simulink model "hierarchical_controller"  (R2025b)
settings: Solver=VariableStepAuto  StartTime=0.0  StopTime=30.0  RelTol=1e-3
InitFcn:
  | %% INITIALIZATION
  | 
  | clearvars -except out
  | clc
  | 
  | %% UAV PARAMETERS
  | 
  | mass = 1.2;        % [kg] mass used by controllers
  | mass_real = 1.2;  % [kg] mass used by dynamics
  | 
  | Ib = diag([1.2416 1.2416 2*1.2416]);
  | Ib_ctrl = diag([1.0 0.85 1.80]);
  | %Ib_ctrl = diag([1.2416 1.2416 2*1.2416]);
  | %% SAMPLING TIME
  | 
  | Ts = 0.001;
  | 
  | %% PLANNER
  | 
  | t_iniz = 0;
  | ttot = 22;       % trajectory duration [s]
  | tdead = 8;       % final steady-state time [s]
  | tot_time = ttot + tdead;
  | 
  | % Include exactly t = ttot
  | t1 = 0:Ts:ttot;
  | t_dead = (ttot+Ts):Ts:tot_time;
  | t = [t1, t_dead];
  | 
  | N1 = length(t1);
  | Ndead = length(t_dead);
  | 
  | %% INITIAL CONDITIONS
  | 
  | x0 = 0;
  | y0 = 0;
  | z0 = -1;
  | psi0 = 0;
  | 
  | x0_real = x0;
  | y0_real = y0;
  | z0_real = z0;
  | 
  | pos_0 = [x0_real y0_real z0_real];
  | lin_vel_0 = [0 0 0];
  | w_bb_0 = [0 0 0];
  | 
  | %% SMOOTH NORMALIZED TIME
  | 
  | sigma = t1 / ttot;
  | 
  | % 7th-order smooth step:
  | % s(0)=0, s(1)=1
  | % sdot(0)=sdot(1)=0
  | % sddot(0)=sddot(1)=0
  | % sdddot(0)=sdddot(1)=0
  | 
  | s = 35*sigma.^4 - 84*sigma.^5 + 70*sigma.^6 - 20*sigma.^7;
  | 
  | sdot = (140*sigma.^3 ...
  |       - 420*sigma.^4 ...
  |       + 420*sigma.^5 ...
  |       - 140*sigma.^6) / ttot;
  | 
  | sddot = (420*sigma.^2 ...
  |        - 1680*sigma.^3 ...
  |        + 2100*sigma.^4 ...
  |        - 840*sigma.^5) / ttot^2;
  | 
  | %% DESIRED TRAJECTORY PARAMETERS
  | 
  | Dx = 1.20;
  | Dy = 0.70;
  | Dz = -1.70;
  | 
  | Ay_bump = 0.35;
  | Az_bump = 0.18;
  | 
  | psi_final = deg2rad(25);
  | psi_bump  = deg2rad(6);
  | 
  | %% DESIRED POSITION
  | 
  | x_d = x0 + Dx*s;
  | 
  | y_d = y0 + Dy*s + Ay_bump*sin(2*pi*s);
  | 
  | z_d = z0 + Dz*s + Az_bump*sin(pi*s);
  | 
  | psi_d_traj = psi0 + psi_final*s + psi_bump*sin(pi*s);
  | 
  | %% DERIVATIVES WITH RESPECT TO s
  | 
  | x_s = Dx;
  | x_ss = 0;
  | 
  | y_s = Dy + Ay_bump*2*pi*cos(2*pi*s);
  | y_ss = -Ay_bump*(2*pi)^2*sin(2*pi*s);
  | 
  | z_s = Dz + Az_bump*pi*cos(pi*s);
  | z_ss = -Az_bump*pi^2*sin(pi*s);
  | 
  | psi_s = psi_final + psi_bump*pi*cos(pi*s);
  | psi_ss = -psi_bump*pi^2*sin(pi*s);
  | 
  | %% DESIRED VELOCITY
  | 
  | dot_x_d = x_s .* sdot;
  | dot_y_d = y_s .* sdot;
  | dot_z_d = z_s .* sdot;
  | 
  | dot_psi_d_traj = psi_s .* sdot;
  | 
  | %% DESIRED ACCELERATION
  | 
  | ddot_x_d = x_ss .* sdot.^2 + x_s .* sddot;
  | ddot_y_d = y_ss .* sdot.^2 + y_s .* sddot;
  | ddot_z_d = z_ss .* sdot.^2 + z_s .* sddot;
  | 
  | ddot_psi_d_traj = psi_ss .* sdot.^2 + psi_s .* sddot;
  | 
  | %% ADD FINAL STEADY-STATE PART
  | 
  | x_final = x_d(end);
  | y_final = y_d(end);
  | z_final = z_d(end);
  | psi_final_value = psi_d_traj(end);
  | 
  | p_d = zeros(4, length(t));
  | dot_p_d = zeros(4, length(t));
  | ddot_p_d = zeros(4, length(t));
  | 
  | p_d(1,:) = [x_d, x_final*ones(1, Ndead)];
  | p_d(2,:) = [y_d, y_final*ones(1, Ndead)];
  | p_d(3,:) = [z_d, z_final*ones(1, Ndead)];
  | p_d(4,:) = [psi_d_traj, psi_final_value*ones(1, Ndead)];
  | 
  | dot_p_d(1,:) = [dot_x_d, zeros(1, Ndead)];
  | dot_p_d(2,:) = [dot_y_d, zeros(1, Ndead)];
  | dot_p_d(3,:) = [dot_z_d, zeros(1, Ndead)];
  | dot_p_d(4,:) = [dot_psi_d_traj, zeros(1, Ndead)];
  | 
  | ddot_p_d(1,:) = [ddot_x_d, zeros(1, Ndead)];
  | ddot_p_d(2,:) = [ddot_y_d, zeros(1, Ndead)];
  | ddot_p_d(3,:) = [ddot_z_d, zeros(1, Ndead)];
  | ddot_p_d(4,:) = [ddot_psi_d_traj, zeros(1, Ndead)];
  | 
  | %% DATA FOR SIMULINK
  | 
  | csi_d = p_d(1:3,:);
  | dot_csi_d = dot_p_d(1:3,:);
  | ddot_csi_d = ddot_p_d(1:3,:);
  | 
  | psi_d = p_d(4,:);
  | dot_psi_d = dot_p_d(4,:);
  | ddot_psi_d = ddot_p_d(4,:);
  | 
  | %% DESIRED BODY X-AXIS FROM YAW
  | 
  | xb_des = zeros(3, length(t));
  | 
  | xb_des(1,:) = cos(psi_d);
  | xb_des(2,:) = sin(psi_d);
  | xb_des(3,:) = zeros(1, length(t));
  | 
  | %% EXTERNAL FORCE DISTURBANCE
  | 
  | f_ext = zeros(length(t), 3);
  | 
  | t_f_on = 8;
  | t_f_off = 14;
  | 
  | f_ex_amp = 1.0;    % [N]
  | f_ey_amp = 1.0;    % [N]
  | f_ez_amp = 0.0;    % [N]
  | 
  | t_smooth_f = 0.3;  % [s] smoothing time
  | 
  | w_on_f  = 0.5 * (1 + tanh((t - t_f_on)/t_smooth_f));
  | w_off_f = 0.5 * (1 - tanh((t - t_f_off)/t_smooth_f));
  | 
  | dist_window_f = w_on_f .* w_off_f;
  | 
  | f_ext(:,1) = f_ex_amp * dist_window_f(:);
  | f_ext(:,2) = f_ey_amp * dist_window_f(:);
  | f_ext(:,3) = f_ez_amp * dist_window_f(:);
  | 
  | f_ext_ts = timeseries(f_ext, t(:));
  | 
  | %% EXTERNAL TORQUE DISTURBANCE
  | 
  | tau_ext = zeros(length(t), 3);
  | 
  | t_tau_on = 8;
  | t_tau_off = 14;
  | 
  | tau_ex_amp = 0.0;    % [Nm]
  | tau_ey_amp = 0.5;    % [Nm]
  | tau_ez_amp = 0.0;    % [Nm]
  | 
  | t_smooth_tau = 0.3;  % [s] smoothing time
  | 
  | w_on_tau  = 0.5 * (1 + tanh((t - t_tau_on)/t_smooth_tau));
  | w_off_tau = 0.5 * (1 - tanh((t - t_tau_off)/t_smooth_tau));
  | 
  | dist_window_tau = w_on_tau .* w_off_tau;
  | 
  | tau_ext(:,1) = tau_ex_amp * dist_window_tau(:);
  | tau_ext(:,2) = tau_ey_amp * dist_window_tau(:);
  | tau_ext(:,3) = tau_ez_amp * dist_window_tau(:);
  | 
  | tau_ext_ts = timeseries(tau_ext, t(:));
  | 
  | 
  | %% CHECK
  | 
  | disp("InitFcn completed.")
  | disp("mass = " + string(mass) + " kg")
  | disp("mass_real = " + string(mass_real) + " kg")
  | disp("Simulation time = " + string(tot_time) + " s")
  | disp("Force disturbance: [" + string(f_ex_amp) + ", " + string(f_ey_amp) + ", " + string(f_ez_amp) + "] N")
  | disp("Torque disturbance: [" + string(tau_ex_amp) + ", " + string(tau_ey_amp) + ", " + string(tau_ez_amp) + "] Nm")
libraries: robotcorelib x1
settings Model: Creator=fabioruggiero  LastModifiedBy=miche
settings ModelReferenceCC: EnableRefExpFcnMdlSchedulingChecks=on
settings RTWCC: GPUComputeCapability=3.5

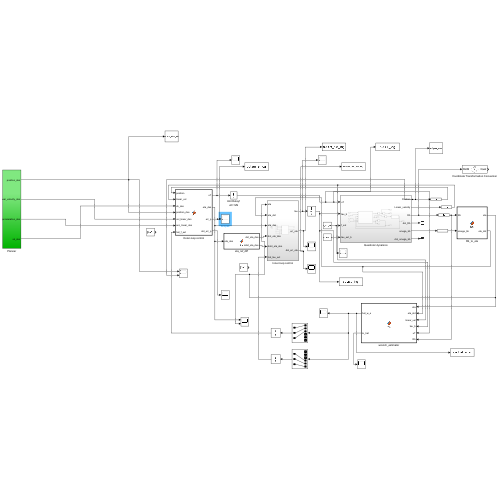
[thumbnail: Simulink's stored preview of the top-level diagram]
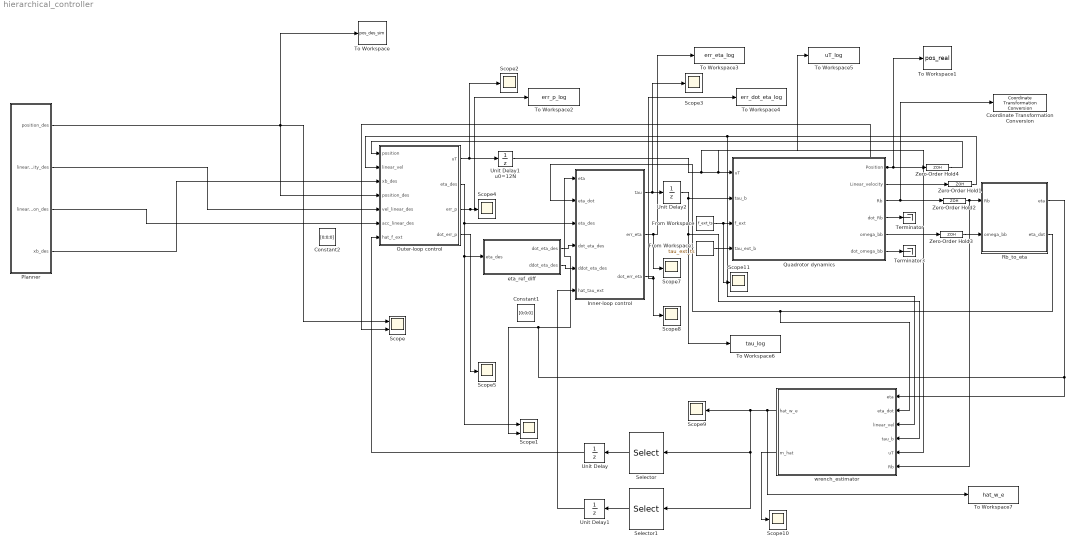
== system hierarchical_controller ==
  Constant1 : Constant  Value=[0;0;0]
  Constant2 : Constant  Value=[0;0;0]
  Coordinate Transformation Conversion : robotcorelib/Coordinate Transformation Conversion  InputRepresentation=Rotation Matrix  InputEulerSequence=ZYX  ShowTrVecInputPort=on  OutputRepresentation=Quaternion  OutputEulerSequence=ZYX  ShowTrVecOutputPort=on  SimulateUsing=Interpreted execution
  From Workspace : FromWorkspace  VariableName=f_ext_ts
  From Workspace1 : FromWorkspace  VariableName=tau_ext_ts
  Inner-loop control : Subsystem
  Outer-loop control : MATLAB Function  TreatAsAtomicUnit=on
  Planner : Subsystem
  Quadrotor dynamics : Subsystem
  Rb_to_eta : MATLAB Function  TreatAsAtomicUnit=on
  Scope : Scope  NumInputPorts=2
      settings: ActiveDisplayYMinimum=-4.8250002447828013  ActiveDisplayYMaximum=3.4250000522047972
  Scope1 : Scope  NumInputPorts=2
      settings: ActiveDisplayYMinimum=-1  ActiveDisplayYMaximum=1
  Scope{2..5,7..11} (9 alike) : Scope
      Scope10 settings: ActiveDisplayYMinimum=1.0530751929618971  ActiveDisplayYMaximum=1.5207401244876457  DataLoggingVariableName=ScopeData11
      Scope11 settings: ActiveDisplayYMinimum=-1  ActiveDisplayYMaximum=1  DataLoggingVariableName=ScopeData12
      Scope2 settings: ActiveDisplayYMinimum=-1  ActiveDisplayYMaximum=1  DataLoggingVariableName=ScopeData2
      Scope3 settings: ActiveDisplayYMinimum=-835.01616147047889  ActiveDisplayYMaximum=458.79322442296439  DataLoggingVariableName=ScopeData3
      Scope4 settings: ActiveDisplayYMinimum=-0.020825285520524945  ActiveDisplayYMaximum=0.020902843774846348  DataLoggingVariableName=ScopeData5
      Scope5 settings: ActiveDisplayYMinimum=-0.31823529054964583  ActiveDisplayYMaximum=0.47295316972389595  DataLoggingVariableName=ScopeData6
      Scope7 settings: ActiveDisplayYMinimum=-1.0945297634041165  ActiveDisplayYMaximum=3.6122729221446721  DataLoggingVariableName=ScopeData8
      Scope8 settings: ActiveDisplayYMinimum=-1  ActiveDisplayYMaximum=1  DataLoggingVariableName=ScopeData9
      Scope9 settings: ActiveDisplayYMinimum=-0.027096582933933789  ActiveDisplayYMaximum=0.033108295929510506  DataLoggingVariableName=ScopeData10
  Selector : Selector  InputPortWidth=6  IndexOptions=Index vector (dialog)  Indices=[1 2 3]  OutputSizes=1
  Selector1 : Selector  InputPortWidth=6  IndexOptions=Index vector (dialog)  Indices=[4 5 6]  OutputSizes=1
  Terminator : Terminator
  Terminator3 : Terminator
  To Workspace : ToWorkspace  VariableName=pos_des_sim  SaveFormat=Timeseries  SampleTime=-1
      settings: Save2DSignal=2-D array (concatenate along first dimension)
  To Workspace1 : ToWorkspace  VariableName=pos_real  SaveFormat=Timeseries  SampleTime=-1
      settings: Save2DSignal=2-D array (concatenate along first dimension)
  To Workspace2 : ToWorkspace  VariableName=err_p_log  SaveFormat=Timeseries  SampleTime=Ts
  To Workspace3 : ToWorkspace  VariableName=err_eta_log  SaveFormat=Timeseries  SampleTime=Ts
  To Workspace4 : ToWorkspace  VariableName=err_dot_eta_log  SaveFormat=Timeseries  SampleTime=Ts
  To Workspace5 : ToWorkspace  VariableName=uT_log  SaveFormat=Timeseries  SampleTime=Ts
  To Workspace6 : ToWorkspace  VariableName=tau_log  SaveFormat=Timeseries  SampleTime=Ts
  To Workspace7 : ToWorkspace  VariableName=hat_w_e  SaveFormat=Timeseries  SampleTime=Ts
  Unit Delay : UnitDelay  InitialCondition=[0; 0; 0]  SampleTime=-1  HasFrameUpgradeWarning=on
  Unit Delay1 : UnitDelay  InitialCondition=[0; 0; 0]  SampleTime=-1  HasFrameUpgradeWarning=on
  Unit Delay1 u0=12N : UnitDelay  InitialCondition=12  SampleTime=Ts
  Unit Delay2 : UnitDelay  InitialCondition=[0;0;0]  SampleTime=Ts
  Zero-Order Hold{1..4} (4 alike) : ZeroOrderHold  SampleTime=Ts
  eta_ref_diff : MATLAB Function  TreatAsAtomicUnit=on
  wrench_estimator : MATLAB Function  TreatAsAtomicUnit=on
  wires:
  Outer-loop control/1(uT) -> Unit Delay1 u0=12N/1, Scope2/1
  Quadrotor dynamics/1(Position) -> Scope/2, To Workspace1/1, Zero-Order Hold4/1
  Quadrotor dynamics/2(Linear_velocity) -> Zero-Order Hold1/1
  Quadrotor dynamics/3(Rb) -> Zero-Order Hold2/1, Coordinate Transformation Conversion/1
  Quadrotor dynamics/5(omega_bb) -> Zero-Order Hold3/1
  Zero-Order Hold2/1 -> wrench_estimator/6(Rb), Rb_to_eta/1(Rb)
  Unit Delay2/1 -> To Workspace6/1, wrench_estimator/4(tau_b), Quadrotor dynamics/2(tau_b)
  Quadrotor dynamics/4(dot_Rb) -> Terminator/1
  Planner/4(xb_des) -> Outer-loop control/3(xb_des)
  Quadrotor dynamics/6(dot_omega_bb) -> Terminator3/1
  Zero-Order Hold3/1 -> Rb_to_eta/2(omega_bb)
  Inner-loop control/1(tau) -> Scope3/1, Unit Delay2/1
  Planner/2(linear_velocity_des) -> Outer-loop control/5(vel_linear_des)
  Planner/3(linear_acceleration_des) -> Outer-loop control/6(acc_linear_des)
  Zero-Order Hold1/1 -> Outer-loop control/2(linear_vel), wrench_estimator/3(linear_vel)
  Zero-Order Hold4/1 -> Outer-loop control/1(position)
  Rb_to_eta/1(eta) -> wrench_estimator/1(eta), Scope1/2, Inner-loop control/1(eta)
  Rb_to_eta/2(eta_dot) -> wrench_estimator/2(eta_dot), Inner-loop control/2(eta_dot)
  Outer-loop control/2(eta_des) -> eta_ref_diff/1(eta_des), Scope1/1, Inner-loop control/3(eta_des)
  eta_ref_diff/1(dot_eta_des) -> Inner-loop control/4(dot_eta_des)
  eta_ref_diff/2(ddot_eta_des) -> Inner-loop control/5(ddot_eta_des)
  Outer-loop control/4(dot_err_p) -> Scope5/1
  Outer-loop control/3(err_p) -> To Workspace2/1, Scope4/1
  Inner-loop control/2(err_eta) -> Scope7/1, To Workspace3/1
  Inner-loop control/3(dot_err_eta) -> To Workspace4/1, Scope8/1
  Planner/1(position_des) -> Outer-loop control/4(position_des), Scope/1, To Workspace/1
  Unit Delay1 u0=12N/1 -> To Workspace5/1, wrench_estimator/5(uT), Quadrotor dynamics/1(uT)
  wrench_estimator/2(m_hat) -> Scope10/1
  wrench_estimator/1(hat_w_e) -> To Workspace7/1, Selector1/1, Selector/1, Scope9/1
  From Workspace/1 -> Scope11/1, Quadrotor dynamics/3(f_ext)
  Selector/1 -> Unit Delay/1
  From Workspace1/1 -> Quadrotor dynamics/4(tau_ext_b)
  Selector1/1 -> Unit Delay1/1
  Unit Delay/1 -> Outer-loop control/7(hat_f_ext)
  Unit Delay1/1 -> Inner-loop control/6(hat_tau_ext)

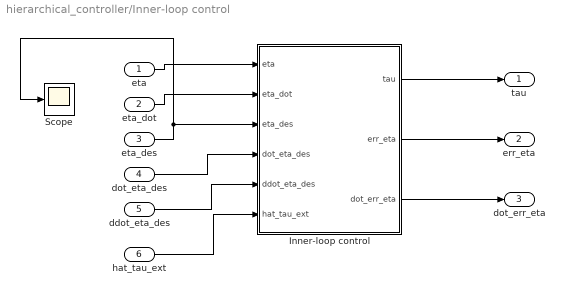
== system hierarchical_controller/Inner-loop control ==
  eta : Inport  PortDimensions=[3 1]
  eta_dot : Inport  Port=2  PortDimensions=[3 1]
  eta_des : Inport  Port=3  PortDimensions=[3 1]
  dot_eta_des : Inport  Port=4  PortDimensions=[3 1]
  ddot_eta_des : Inport  Port=5  PortDimensions=[3 1]
  hat_tau_ext : Inport  Port=6
  Inner-loop control : MATLAB Function  TreatAsAtomicUnit=on
  Scope : Scope
      settings: ActiveDisplayYMinimum=-1  ActiveDisplayYMaximum=1  DataLoggingVariableName=ScopeData4
  tau : Outport
  err_eta : Outport  Port=2  PortDimensions=[3 1]
  dot_err_eta : Outport  Port=3
  wires:
  dot_eta_des/1 -> Inner-loop control/4(dot_eta_des)
  Inner-loop control/2(err_eta) -> err_eta/1
  eta_dot/1 -> Inner-loop control/2(eta_dot)
  Inner-loop control/1(tau) -> tau/1
  Inner-loop control/3(dot_err_eta) -> dot_err_eta/1
  eta/1 -> Inner-loop control/1(eta)
  eta_des/1 -> Scope/1, Inner-loop control/3(eta_des)
  ddot_eta_des/1 -> Inner-loop control/5(ddot_eta_des)
  hat_tau_ext/1 -> Inner-loop control/6(hat_tau_ext)

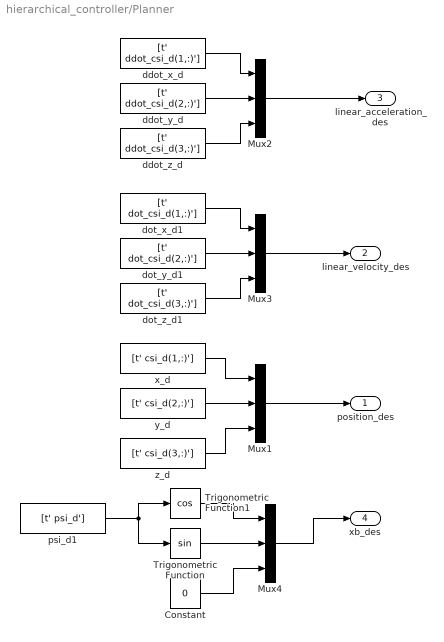
== system hierarchical_controller/Planner ==
  Constant : Constant  Value=0
  Mux{1..4} (4 alike) : Mux  Inputs=3
  Trigonometric Function : Trigonometry
  Trigonometric Function1 : Trigonometry  Operator=cos
  ddot_x_d : FromWorkspace  VariableName=[t' ddot_csi_d(1,:)']  SampleTime=Ts
  ddot_y_d : FromWorkspace  VariableName=[t' ddot_csi_d(2,:)']  SampleTime=Ts
  ddot_z_d : FromWorkspace  VariableName=[t' ddot_csi_d(3,:)']  SampleTime=Ts
  dot_x_d1 : FromWorkspace  VariableName=[t' dot_csi_d(1,:)']  SampleTime=Ts
  dot_y_d1 : FromWorkspace  VariableName=[t' dot_csi_d(2,:)']  SampleTime=Ts
  dot_z_d1 : FromWorkspace  VariableName=[t' dot_csi_d(3,:)']  SampleTime=Ts
  psi_d1 : FromWorkspace  VariableName=[t' psi_d']  SampleTime=Ts
  x_d : FromWorkspace  VariableName=[t' csi_d(1,:)']  SampleTime=Ts
  y_d : FromWorkspace  VariableName=[t' csi_d(2,:)']  SampleTime=Ts
  z_d : FromWorkspace  VariableName=[t' csi_d(3,:)']  SampleTime=Ts
  position_des : Outport
  linear_velocity_des : Outport  Port=2
  linear_acceleration_des : Outport  Port=3
  xb_des : Outport  Port=4
  wires:
  y_d/1 -> Mux1/2
  z_d/1 -> Mux1/3
  x_d/1 -> Mux1/1
  ddot_y_d/1 -> Mux2/2
  ddot_z_d/1 -> Mux2/3
  ddot_x_d/1 -> Mux2/1
  Mux2/1 -> linear_acceleration_des/1
  Mux1/1 -> position_des/1
  dot_y_d1/1 -> Mux3/2
  dot_z_d1/1 -> Mux3/3
  dot_x_d1/1 -> Mux3/1
  Mux3/1 -> linear_velocity_des/1
  Mux4/1 -> xb_des/1
  Trigonometric Function/1 -> Mux4/2
  psi_d1/1 -> Trigonometric Function/1, Trigonometric Function1/1
  Trigonometric Function1/1 -> Mux4/1
  Constant/1 -> Mux4/3

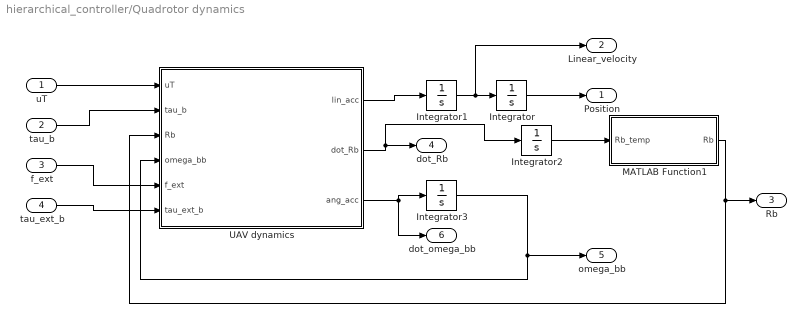
== system hierarchical_controller/Quadrotor dynamics ==
  uT : Inport
  tau_b : Inport  Port=2
  f_ext : Inport  Port=3
  tau_ext_b : Inport  Port=4
  Integrator : Integrator  InitialCondition=pos_0
  Integrator1 : Integrator  InitialCondition=lin_vel_0
  Integrator2 : Integrator  InitialCondition=[1 0 0; 0 1 0;0 0 1]
  Integrator3 : Integrator  InitialCondition=w_bb_0
  MATLAB Function1 : MATLAB Function  TreatAsAtomicUnit=on
  UAV dynamics : MATLAB Function  TreatAsAtomicUnit=on
  Position : Outport
  Linear_velocity : Outport  Port=2
  Rb : Outport  Port=3
  dot_Rb : Outport  Port=4
  omega_bb : Outport  Port=5
  dot_omega_bb : Outport  Port=6
  wires:
  tau_b/1 -> UAV dynamics/2(tau_b)
  Integrator/1 -> Position/1
  UAV dynamics/3(ang_acc) -> Integrator3/1, dot_omega_bb/1
  UAV dynamics/1(lin_acc) -> Integrator1/1
  uT/1 -> UAV dynamics/1(uT)
  Integrator1/1 -> Linear_velocity/1, Integrator/1
  Integrator3/1 -> UAV dynamics/4(omega_bb), omega_bb/1
  UAV dynamics/2(dot_Rb) -> Integrator2/1, dot_Rb/1
  MATLAB Function1/1(Rb) -> Rb/1, UAV dynamics/3(Rb)
  Integrator2/1 -> MATLAB Function1/1(Rb_temp)
  f_ext/1 -> UAV dynamics/5(f_ext)
  tau_ext_b/1 -> UAV dynamics/6(tau_ext_b)

== matlab function hierarchical_controller/Rb_to_eta ==
  data: Rb input; eta output; omega_bb input; eta_dot output
function [eta, eta_dot] = fcn(Rb, omega_bb)

r31 = Rb(3,1);
r31 = max(min(r31,1),-1);

phi   = atan2(Rb(3,2), Rb(3,3));
theta = -asin(r31);
psi   = atan2(Rb(2,1), Rb(1,1));

eta = [phi; theta; psi];

cphi = cos(phi);
sphi = sin(phi);
cth  = cos(theta);
sth  = sin(theta);

Q = [1, 0, -sth;
     0, cphi, cth*sphi;
     0, -sphi, cth*cphi];

eta_dot = Q \ omega_bb;

== matlab function hierarchical_controller/Quadrotor dynamics/UAV dynamics ==
  data: uT input size=1; tau_b input size=3; lin_acc output size=3; Rb input size=[3,3]; omega_bb input size=3; dot_Rb output size=[3,3]; ang_acc output size=3; mass parameter size=1; Ib parameter size=[3,3]; f_ext input; tau_ext_b input
function [lin_acc, dot_Rb, ang_acc] = fcn(uT, tau_b, Rb, omega_bb, mass, Ib, f_ext, tau_ext_b)

tau_b = reshape(tau_b, [3 1]);
tau_ext_b = reshape(tau_ext_b, [3 1]);
omega_bb = reshape(omega_bb, [3 1]);
Rb = reshape(Rb, [3 3]);
Ib = reshape(Ib, [3 3]);
f_ext = reshape(f_ext, [3 1]);

e3 = [0; 0; 1];
g = 9.81;

% Translational dynamics with external force
lin_acc = g*e3 - (uT/mass)*Rb*e3 + f_ext/mass;

% Rotational dynamics with external body torque
dot_Rb = Rb * skew(omega_bb);

ang_acc = Ib \ (-skew(omega_bb)*Ib*omega_bb + tau_b + tau_ext_b);

end


function S = skew(v)

v = reshape(v, [3 1]);

S = [   0   -v(3)  v(2);
      v(3)    0   -v(1);
     -v(2)  v(1)    0];

end

== matlab function hierarchical_controller/Outer-loop control ==
  data: position input size=3; uT output size=1; linear_vel input size=3; xb_des input size=[3,1]; eta_des output size=3; position_des input size=3; vel_linear_des input size=3; acc_linear_des input size=3; err_p output size=3; dot_err_p output size=3; hat_f_ext input
function [uT, eta_des, err_p, dot_err_p] = fcn(position, linear_vel, xb_des, ...
    position_des, vel_linear_des, acc_linear_des, hat_f_ext)

% mass is taken from workspace (InitFcn)
g = 9.81;
mass = 1.2;

% gains
Kp = diag([12 12 12]);
Kv = diag([6 6 6]);

% errors
err_p = position - position_des;
dot_err_p = linear_vel - vel_linear_des;

hat_f_ext = reshape(hat_f_ext, [3 1]);

% nominal virtual input
mu_d_nom = -Kp*err_p - Kv*dot_err_p + acc_linear_des;

% external force compensation
mu_d = mu_d_nom - hat_f_ext/mass;

mu_x = mu_d(1);
mu_y = mu_d(2);
mu_z = mu_d(3);

% yaw desired from xb_des
psi_des = atan2(xb_des(2), xb_des(1));

% thrust
uT = mass * sqrt(mu_x^2 + mu_y^2 + (mu_z - g)^2);
uT = max(uT, 1e-6);

% desired roll and pitch
arg_phi = (mass/uT) * (mu_y*cos(psi_des) - mu_x*sin(psi_des));
arg_phi = max(min(arg_phi,1),-1);

phi_d = asin(arg_phi);
theta_d = atan2((mu_x*cos(psi_des) + mu_y*sin(psi_des)), (mu_z - g));
theta_d = atan2(-(mu_x*cos(psi_des) + mu_y*sin(psi_des)), (g - mu_z));

eta_des = [phi_d; theta_d; psi_des];

== matlab function hierarchical_controller/Inner-loop control/Inner-loop control ==
  data: tau output size=[3,1]; err_eta output size=[3,1]; dot_err_eta output size=[3,1]; eta input size=[3,1]; eta_dot input size=[3,1]; eta_des input size=[3,1]; dot_eta_des input size=[3,1]; ddot_eta_des input size=[3,1]; hat_tau_ext input
function [tau, err_eta, dot_err_eta] = fcn(eta, eta_dot, eta_des, dot_eta_des, ddot_eta_des, hat_tau_ext)

Ts = 0.001;
Ib = diag([1.2416 1.2416 2*1.2416]);

% Force column vectors
eta          = reshape(eta,          [3 1]);
eta_dot      = reshape(eta_dot,      [3 1]);
eta_des      = reshape(eta_des,      [3 1]);
dot_eta_des  = reshape(dot_eta_des,  [3 1]);
ddot_eta_des = reshape(ddot_eta_des, [3 1]);
hat_tau_ext  = reshape(hat_tau_ext,  [3 1]);

% Force output sizes for Simulink inference
tau         = zeros(3,1);
err_eta     = zeros(3,1);
dot_err_eta = zeros(3,1);

% Gains
K1 = diag([10 10 8]);
K2 = diag([6 6 5]);

% Errors
err_eta(:) = eta - eta_des;
dot_err_eta(:) = eta_dot - dot_eta_des;

% Matrices
Q = Q_matrix(eta);
C = C_matrix(eta, eta_dot, Ts, Ib);

% Nominal inner-loop control
tau_tilde = -K1*err_eta - K2*dot_err_eta + ddot_eta_des;

tau_nom = Ib * Q * tau_tilde + (Q') \ (C * eta_dot);

% External generalized torque compensation
% hat_tau_ext = hat_w_e(4:6) is in generalized RPY coordinates.
% Convert compensation to body torque:
tau_comp = -(Q') \ hat_tau_ext;

% Final torque command
tau(:) = tau_nom + tau_comp;

end


function Q = Q_matrix(eta)

eta = reshape(eta, [3 1]);

phi = eta(1);
theta = eta(2);

cphi = cos(phi);
sphi = sin(phi);
cth  = cos(theta);
sth  = sin(theta);

Q = [1, 0, -sth;
     0, cphi, cth*sphi;
     0, -sphi, cth*cphi];

end


function C = C_matrix(eta, eta_dot, Ts, Ib)

eta     = reshape(eta,     [3 1]);
eta_dot = reshape(eta_dot, [3 1]);

persistent eta_prev
if isempty(eta_prev)
    eta_prev = eta;
end

Q = Q_matrix(eta);
Q_prev = Q_matrix(eta_prev);

Q_dot = (Q - Q_prev)/Ts;
omega = Q * eta_dot;

C = Q' * skew(omega) * Ib * Q + Q' * Ib * Q_dot;

eta_prev = eta;

end


function S = skew(v)

v = reshape(v, [3 1]);

S = [   0   -v(3)  v(2);
      v(3)    0   -v(1);
     -v(2)  v(1)    0];

end

== matlab function hierarchical_controller/Quadrotor dynamics/MATLAB Function1 ==
  data: Rb_temp input; Rb output
function Rb = fcn(Rb_temp)
    [U,S,V] = svd(Rb_temp);
    sigma = det(U*V');
    S_ = diag([1 1 sigma]);

    Rb = U*S_*V';
end

== matlab function hierarchical_controller/eta_ref_diff ==
  data: eta_des input; dot_eta_des output; ddot_eta_des output
function [dot_eta_des, ddot_eta_des] = fcn(eta_des)

Ts = 0.001;

eta_des = reshape(eta_des, [3 1]);

persistent eta_des_prev dot_eta_des_prev initialized

if isempty(initialized)
    eta_des_prev = eta_des;
    dot_eta_des_prev = zeros(3,1);
    initialized = true;
end

dot_eta_des = (eta_des - eta_des_prev) / Ts;

ddot_eta_des = (dot_eta_des - dot_eta_des_prev) / Ts;

eta_des_prev = eta_des;
dot_eta_des_prev = dot_eta_des;

end

== matlab function hierarchical_controller/wrench_estimator ==
  data: eta input; hat_w_e output; eta_dot input; linear_vel input; tau_b input; uT input; Rb input; m_hat output
function [hat_w_e, m_hat] = fcn(eta, eta_dot, linear_vel, tau_b, uT, Rb)

% External wrench estimator
% hat_w_e = [f_ext_world; tau_ext_generalized]

Ts = 0.001;

m = 1.2;
J = diag([1.2416 1.2416 2*1.2416]);
g = 9.81;
e3 = [0; 0; 1];

% ==========================
% Estimator parameters
% ==========================
r = 3;           % try: 1, 2, 3, 5, 10
omega_c = 12;    % cutoff frequency [rad/s]

RMAX = 20;
r = max(1, min(round(r), RMAX));

% ==========================
% Compute gains K from (s + omega_c)^r
% ==========================
K = zeros(1, RMAX);
c = zeros(1, RMAX);

for j = 0:RMAX-1
    if j <= r-1
        c(j+1) = binom_coeff(r,j) * omega_c^(r-j);
    end
end

K(r) = c(r);

for j = RMAX-1:-1:1
    if j < r
        prod_next = 1;
        for k = j+1:r
            prod_next = prod_next * K(k);
        end
        K(j) = c(j) / prod_next;
    end
end

% ==========================
% Force dimensions
% ==========================
eta        = reshape(eta,        [3 1]);
eta_dot    = reshape(eta_dot,    [3 1]);
linear_vel = reshape(linear_vel, [3 1]);
tau_b      = reshape(tau_b,      [3 1]);
Rb         = reshape(Rb,         [3 3]);

hat_w_e = zeros(6,1);
m_hat = 0;

persistent gamma hat_w_prev int_hat_w int_model eta_prev initialized

if isempty(initialized)
    gamma = zeros(6, RMAX);
    hat_w_prev = zeros(6,1);
    int_hat_w = zeros(6,1);
    int_model = zeros(6,1);
    eta_prev = eta;
    initialized = true;
end

% ==========================
% Model matrices
% ==========================
Q = Q_matrix(eta);
C = C_matrix(eta, eta_dot, eta_prev, Ts, J);
M_eta = Q' * J * Q;

% Generalized momentum
q = [m*eye(3), zeros(3,3);
     zeros(3,3), M_eta] * [linear_vel; eta_dot];

% Nominal model term
upper = m*g*e3 - uT * Rb * e3;
lower = C' * eta_dot + Q' * tau_b;

model_term = [upper; lower];

% ==========================
% Integrals
% ==========================
int_hat_w = int_hat_w + hat_w_prev * Ts;
int_model = int_model + model_term * Ts;

% ==========================
% r-th order estimator
% ==========================
gamma(:,1) = K(1) * (q - int_hat_w - int_model);

for i = 2:RMAX
    if i <= r
        gamma(:,i) = gamma(:,i) + ...
            K(i) * (gamma(:,i-1) - hat_w_prev) * Ts;
    end
end

hat_w_e = gamma(:,r);
hat_w_prev = hat_w_e;

% Mass estimate
m_hat = (uT * Rb(3,:) * e3 - hat_w_e(3)) / g;

eta_prev = eta;

end


function Q = Q_matrix(eta)

phi = eta(1);
theta = eta(2);

cphi = cos(phi);
sphi = sin(phi);
cth  = cos(theta);
sth  = sin(theta);

Q = [1, 0, -sth;
     0, cphi, cth*sphi;
     0, -sphi, cth*cphi];

end


function C = C_matrix(eta, eta_dot, eta_prev, Ts, J)

Q = Q_matrix(eta);
Q_prev = Q_matrix(eta_prev);

Q_dot = (Q - Q_prev) / Ts;
omega = Q * eta_dot;

C = Q' * skew(omega) * J * Q + Q' * J * Q_dot;

end


function S = skew(v)

v = reshape(v, [3 1]);

S = [   0   -v(3)  v(2);
      v(3)    0   -v(1);
     -v(2)  v(1)    0];

end


function b = binom_coeff(n,k)

b = 1;

if k < 0 || k > n
    b = 0;
else
    for i = 1:k
        b = b * (n - k + i) / i;
    end
end

end
